simulink model "mfordmodel_v1"  (R2023a)
settings: Solver=ode45  StartTime=0.0  StopTime=10.0  RelTol=1e-3  EnableMultiTasking=on
undefined symbols (not defined in the file): ABV_RATIO_SW, AC_OFF_DLY, ACLOD, AUTO_TRNS_SW, BRAKE_DNDT_X, BZZRPM, BZZRPM_ALT, BZZTM, BZZTM_ALT, CMD_LITOFF, CMD_STABLE, CO_ST_ECT__A, COOL_BASE, DAS_BKDLY_A, DAS_CNT, DAS_CTDLY, DAS_LC_SW__A, DASCLP_5INH, DASCTL, DASMHYST, DASMPH, DEBYCP, DES_BASE, DPNEU_MUL, DSDRPM_DN_TC, DSDRPM_OFF, DSDRPM_UP_TC, EDF_DELAY, EDFHP, ETC_CL_TP, ETC_HP, GR_CM_CREEP, HCAM_ACT_CLP, HEDFHP, HEDFRPM, HICAM_PS, IAC_CAL_SW, IAC_ER_TM1, IAC_ER_TM2, IAC_ER_TM4, IAC_HI_LIM__A, IAC_ISFL_OBD, IAC_KAM_SW, IAC_LO_LIM__A, IAC_MON_TM, IAC_OT_REQ, IAC_RUN_TM, IAC_TP_OBD, IAC_TR_DAS, IAC_TST_DC, ID_DAS__A, ID_NOVS__A, IDVS_CH__A, IDVS_SL__A, IPSI_SW, IPSIDLY, IS_DRBASE__A, IS_DRBASE_A__A, IS_NUBASE__A, IS_NUBASE_A__A ... (+35)
libraries: simulink x2
(part 6 of 12)

== system mfordmodel_v1/iac_v04_001_001/activate_desired_rpm/hicam_rpm_request/isadd_ramp/CONSTANT ==
  Constant : Constant  Value=const
  Out : Outport
  wires:
  Constant/1 -> Out/1

== system mfordmodel_v1/iac_v04_001_001/activate_desired_rpm/hicam_rpm_request/isadd_ramp/ROLAV_TC_in_DT_in ==
  note: Using the first two terms of the series expansion:
      |
      |                     x                     x2
      |                                e   =  1  +  x  +  --  + ......
      |                                           2!
      |
      |       Simplifying, the exponential "f" becomes:
      |
      |                  - (FK_TMR/TC)              1
      |           f  =  1  -  e                    =  1  -  -------------  =  . . .
      |                                                    (FK_TMR/TC)
      |                           e
      |
      |                              1                      1
      |          f  =  1  -  ---------------------------------  =    ------------------- .
      |                                  1 + (FK_TMR / TC)       1 + (TC / FK_TMR)
  note: - (FK_TMR/TC)
      |                                    f  =  1  -  e
      |
      |       Where "f" is called the filter constant in the difference equation:
      |
      |                    new_average = f * new_value + (1 - f) * old_average
  note: new_average = [ (sample_interval)/(sample_interval + time_constant) ] * (new_value - old_ave) + old_ave
  new_value : Inport
  Tau : Inport  Port=2
  old_ave : Inport  Port=3
  delta_time : Inport  Port=4
  Elementary Math : Math  Operator=reciprocal  SignedPower=on
  Product : Product  Inputs=3  InputSameDT=on  RndMeth=Zero  SaturateOnIntegerOverflow=on  OutDataTypeStr=Inherit: Same as first input
  Sum : Sum  Inputs=-+  InputSameDT=on  SaturateOnIntegerOverflow=on  OutDataTypeStr=Inherit: Same as first input
  Sum1 : Sum  InputSameDT=on  SaturateOnIntegerOverflow=on  OutDataTypeStr=Inherit: Same as first input
  Sum2 : Sum  InputSameDT=on  SaturateOnIntegerOverflow=on  OutDataTypeStr=Inherit: Same as first input
  new_ave : Outport
  wires:
  delta_time/1 -> Product/2, Sum1/1
  Tau/1 -> Sum1/2
  Sum2/1 -> new_ave/1
  old_ave/1 -> Sum2/1, Sum/1
  Product/1 -> Sum2/2
  Sum/1 -> Product/1
  Elementary Math/1 -> Product/3
  Sum1/1 -> Elementary Math/1
  new_value/1 -> Sum/2

== system mfordmodel_v1/iac_v04_001_001/iac_executive/fault_code_setting/TIMER_DT_in/Time Calculator ==
  note: Timer Control calls the counters 'delta_time' and 'timer_calculation'
      | after using the flags 'increment_flag' and 'decrement_flag'
      | to determine the direction of the timer.
  note: Increment, hold,
      | or decrement
  note: Resets timer
      | to 'reset_value'
  note: Calculates time
      | between cycles.
      | Activated every cycle.
  note: Calculates timer value.
      | Activated only when
      | counting up or down.
  count_direction : Inport
  reset_val : Inport  Port=2
  do_delta_time : Inport  Port=3
  do_timer : Inport  Port=4
  reset_value : Inport  Port=5
  delta time : Inport  Port=6
  From : From
  Goto : Goto
  delta_time : Subsystem  TreatAsAtomicUnit=on
  timer_calculation : Subsystem  TreatAsAtomicUnit=on
  timer : Outport
  wires:
  do_delta_time/1 -> delta_time/Trigger  "do_delta_time"
  delta_time/1(delta_time) -> Goto/1  "delta_time"
  count_direction/1 -> delta_time/1(count_direction)  "count_direction"
  timer_calculation/1(timer) -> timer/1  "timer"
  From/1 -> timer_calculation/3(delta_time)  "delta_time"
  do_timer/1 -> timer_calculation/Trigger  "do_timer"
  reset_val/1 -> timer_calculation/2(reset_flag)  "reset_flag"
  reset_value/1 -> timer_calculation/1(reset_value)  "reset_value"
  delta time/1 -> delta_time/2(count_direction1)  "delta_time"

== system mfordmodel_v1/iac_v04_001_001/iac_executive/misc_calcs/TIMER_DT_in/Time Calculator ==
  note: Timer Control calls the counters 'delta_time' and 'timer_calculation'
      | after using the flags 'increment_flag' and 'decrement_flag'
      | to determine the direction of the timer.
  note: Increment, hold,
      | or decrement
  note: Resets timer
      | to 'reset_value'
  note: Calculates time
      | between cycles.
      | Activated every cycle.
  note: Calculates timer value.
      | Activated only when
      | counting up or down.
  count_direction : Inport
  reset_val : Inport  Port=2
  do_delta_time : Inport  Port=3
  do_timer : Inport  Port=4
  reset_value : Inport  Port=5
  delta time : Inport  Port=6
  From : From
  Goto : Goto
  delta_time : Subsystem  TreatAsAtomicUnit=on
  timer_calculation : Subsystem  TreatAsAtomicUnit=on
  timer : Outport
  wires:
  do_delta_time/1 -> delta_time/Trigger  "do_delta_time"
  delta_time/1(delta_time) -> Goto/1  "delta_time"
  count_direction/1 -> delta_time/1(count_direction)  "count_direction"
  timer_calculation/1(timer) -> timer/1  "timer"
  From/1 -> timer_calculation/3(delta_time)  "delta_time"
  do_timer/1 -> timer_calculation/Trigger  "do_timer"
  reset_val/1 -> timer_calculation/2(reset_flag)  "reset_flag"
  reset_value/1 -> timer_calculation/1(reset_value)  "reset_value"
  delta time/1 -> delta_time/2(count_direction1)  "delta_time"

== system mfordmodel_v1/iac_v04_001_001/iac_executive/misc_calcs/dndt_calc/ROLAV_TC_DT_in ==
  note: Using the first two terms of the series expansion:
      |
      |                     x                     x2
      |                                e   =  1  +  x  +  --  + ......
      |                                           2!
      |
      |       Simplifying, the exponential "f" becomes:
      |
      |                  - (FK_TMR/TC)              1
      |           f  =  1  -  e                    =  1  -  -------------  =  . . .
      |                                                    (FK_TMR/TC)
      |                           e
      |
      |                              1                      1
      |          f  =  1  -  ---------------------------------  =    ------------------- .
      |                                  1 + (FK_TMR / TC)       1 + (TC / FK_TMR)
  note: - (FK_TMR/TC)
      |                                    f  =  1  -  e
      |
      |       Where "f" is called the filter constant in the difference equation:
      |
      |                    new_average = f * new_value + (1 - f) * old_average
  note: new_average = [ (sample_interval)/(sample_interval + time_constant) ] * (new_value - old_ave) + old_ave
  new_value : Inport
  old_ave : Inport  Port=2
  delta_time : Inport  Port=3
  Elementary Math : Math  Operator=reciprocal  SignedPower=on
  Product : Product  Inputs=3  InputSameDT=on  RndMeth=Zero  SaturateOnIntegerOverflow=on  OutDataTypeStr=Inherit: Same as first input
  Sum : Sum  Inputs=-+  InputSameDT=on  SaturateOnIntegerOverflow=on  OutDataTypeStr=Inherit: Same as first input
  Sum1 : Sum  InputSameDT=on  SaturateOnIntegerOverflow=on  OutDataTypeStr=Inherit: Same as first input
  Sum2 : Sum  InputSameDT=on  SaturateOnIntegerOverflow=on  OutDataTypeStr=Inherit: Same as first input
  Time Constant : Constant  Value=tc
  new_ave : Outport
  wires:
  Time Constant/1 -> Sum1/2
  Sum2/1 -> new_ave/1
  old_ave/1 -> Sum2/1, Sum/1
  Product/1 -> Sum2/2
  Sum/1 -> Product/1
  Elementary Math/1 -> Product/3
  Sum1/1 -> Elementary Math/1
  new_value/1 -> Sum/2
  delta_time/1 -> Product/2, Sum1/1

== system mfordmodel_v1/iac_v04_001_001/iac_executive/mode_control/crank_mode/crank_calcs ==
  ml_flow_sel_sw : Inport
  tcstrt : Inport  Port=2
  ratch : Inport  Port=3
  do_crank_calcs : TriggerPort  TriggerType=function-call  VariantControl=(inherit)
  Constant : Constant  Value=0.0
  Constant1 : Constant  Value=0.0
  Constant2 : Constant
  Gain : Gain  SaturateOnIntegerOverflow=on  OutDataTypeStr=Inherit: Same as input  ParamDataTypeStr=Inherit: Same as input
  ISCFLG_DASHPOT_PREPOSITION : Constant  Value=0
  Multiport Switch9 : MultiPortSwitch  Inputs=2
  lookup_2d FN818 : Subsystem  mask(2-D, piece-wise, linear interpolation){CAL_FUNC=FNCRANK_PPM}
      mask prompts: CAL_FUNC "Calibration function name"
      mask help:
      | Performs piece-wise linear interpolation.
      |
      | Output is NOT extrapolated beyond the input range.  If the input value presented to the block lies outside the range specified in the block's parameter, then the value is treated as though it has the value of the nearest value in the range.
      mask init: same as mfordmodel_v1/iac_v04_001_001/activate_desired_rpm/rpm_calcs/lookup_2d
      mask Help:
      | Enter the name of the calibration function.
      | (e.g. EGM_VA_ECT_MULT)
      mask Display:
      | fprintf('%s',CAL_FUNC);
      | plot(calfunc.X,calfunc.Y,max_x*1.05,max_y*1.05,min_x,min_y);
  abv_ratio : Outport  InitialOutput=[0]
  abv_flowrate : Outport  Port=2  InitialOutput=[0]
  hcamfg : Outport  Port=3  InitialOutput=[0]
  iscflg : Outport  Port=4  InitialOutput=[0]
  dstpbr : Outport  Port=5  InitialOutput=[0]
  wires:
  Gain/1 -> dstpbr/1  "dstpbr"
  ratch/1 -> Gain/1
  ISCFLG_DASHPOT_PREPOSITION/1 -> iscflg/1  "iscflg"
  Constant2/1 -> hcamfg/1  "hcamfg"
  Multiport Switch9/1 -> abv_flowrate/1  "abv_flowrate"
  ml_flow_sel_sw/1 -> Multiport Switch9/1
  lookup_2d FN818/1(Out1) -> Multiport Switch9/2
  tcstrt/1 -> lookup_2d FN818/1(In1)
  Constant1/1 -> Multiport Switch9/3
  Constant/1 -> abv_ratio/1  "abv_ratio"

== system mfordmodel_v1/iac_v04_001_001/iac_executive/mode_control/external_override_mode/flowrate_set ==
  ml_flow_sel_sw : Inport
  abv_flowrate_osc : Inport  Port=2
  abv_flowrate_in : Inport  Port=3
  abv_ratio_in : Inport  Port=4
  do_flowrate_set : TriggerPort  TriggerType=function-call  VariantControl=(inherit)
  Constant4 : Constant  Value=15.99976
  Constant5 : Constant  Value=0.0
  Constant6 : Constant  Value=0.0
  Multiport Switch : MultiPortSwitch  Inputs=4
  Multiport Switch1 : MultiPortSwitch  Inputs=4
  abv_flowrate : Outport
  abv_ratio : Outport  Port=2
  wires:
  abv_ratio_in/1 -> Multiport Switch1/5
  abv_flowrate_in/1 -> Multiport Switch/5
  Constant6/1 -> Multiport Switch1/4, Multiport Switch1/3, Multiport Switch1/2
  ml_flow_sel_sw/1 -> Multiport Switch/1, Multiport Switch1/1
  Multiport Switch1/1 -> abv_ratio/1  "abv_ratio"
  Constant5/1 -> Multiport Switch/4
  Constant4/1 -> Multiport Switch/3
  abv_flowrate_osc/1 -> Multiport Switch/2
  Multiport Switch/1 -> abv_flowrate/1  "abv_flowrate"

== system mfordmodel_v1/iac_v04_001_001/iac_executive/mode_control/external_override_mode/substitute ==
  note: For now, just pass through the value.
      | Later, the substitution logic will be added.
  OSC_in : Inport
  do_substitute : TriggerPort  TriggerType=function-call  VariantControl=(inherit)
  Gain : Gain  SaturateOnIntegerOverflow=on  OutDataTypeStr=Inherit: Same as input  ParamDataTypeStr=Inherit: Same as input
  OSC_out : Outport
  wires:
  Gain/1 -> OSC_out/1
  OSC_in/1 -> Gain/1

== system mfordmodel_v1/iac_v04_001_001/iac_executive/mode_control/failure_mode/CONSTANT1 ==
  Constant : Constant  Value=const
  Out : Outport
  wires:
  Constant/1 -> Out/1

== system mfordmodel_v1/iac_v04_001_001/iac_executive/runup_flag_timer/TIMER_DT_in/Time Calculator ==
  note: Timer Control calls the counters 'delta_time' and 'timer_calculation'
      | after using the flags 'increment_flag' and 'decrement_flag'
      | to determine the direction of the timer.
  note: Increment, hold,
      | or decrement
  note: Resets timer
      | to 'reset_value'
  note: Calculates time
      | between cycles.
      | Activated every cycle.
  note: Calculates timer value.
      | Activated only when
      | counting up or down.
  count_direction : Inport
  reset_val : Inport  Port=2
  do_delta_time : Inport  Port=3
  do_timer : Inport  Port=4
  reset_value : Inport  Port=5
  delta time : Inport  Port=6
  From : From
  Goto : Goto
  delta_time : Subsystem  TreatAsAtomicUnit=on
  timer_calculation : Subsystem  TreatAsAtomicUnit=on
  timer : Outport
  wires:
  do_delta_time/1 -> delta_time/Trigger  "do_delta_time"
  delta_time/1(delta_time) -> Goto/1  "delta_time"
  count_direction/1 -> delta_time/1(count_direction)  "count_direction"
  timer_calculation/1(timer) -> timer/1  "timer"
  From/1 -> timer_calculation/3(delta_time)  "delta_time"
  do_timer/1 -> timer_calculation/Trigger  "do_timer"
  reset_val/1 -> timer_calculation/2(reset_flag)  "reset_flag"
  reset_value/1 -> timer_calculation/1(reset_value)  "reset_value"
  delta time/1 -> delta_time/2(count_direction1)  "delta_time"

== system mfordmodel_v1/iac_v04_001_001/normal_mode/activate_feedforward/ac_ppm_tmr/Time Calculator ==
  note: Calculates timer value.
      | Activated only when
      | counting up or down.
  note: Calculates time
      | between cycles.
      | Activated every cycle.
  note: Resets timer
      | to 'reset_value'
  note: Increment, hold,
      | or decrement
  note: Timer Control calls the counters 'delta_time' and 'timer_calculation'
      | after using the flags 'increment_flag' and 'decrement_flag'
      | to determine the direction of the timer.
  note: timer14/TIMER/Time Calculator
  count_direction : Inport
  reset_val : Inport  Port=2
  do_delta_time : Inport  Port=3
  do_timer : Inport  Port=4
  reset_value : Inport  Port=5
  From : From
  Goto : Goto
  delta_time : Subsystem  TreatAsAtomicUnit=on
  timer_calculation : Subsystem  TreatAsAtomicUnit=on
  timer : Outport
  wires:
  reset_value/1 -> timer_calculation/1(reset_value)  "reset_value"
  reset_val/1 -> timer_calculation/2(reset_flag)  "reset_flag"
  do_timer/1 -> timer_calculation/Trigger  "do_timer"
  From/1 -> timer_calculation/3(delta_time)  "delta_time"
  timer_calculation/1(timer) -> timer/1  "timer"
  count_direction/1 -> delta_time/1(count_direction)  "count_direction"
  delta_time/1(delta_time) -> Goto/1  "delta_time"
  do_delta_time/1 -> delta_time/Trigger  "do_delta_time"

== system mfordmodel_v1/iac_v04_001_001/normal_mode/activate_feedforward/desmaf_pre_calc/   ==
  Constant : Constant  Value=const
  Out : Outport
  wires:
  Constant/1 -> Out/1

== system mfordmodel_v1/iac_v04_001_001/normal_mode/activate_feedforward/desmaf_pre_calc/  2 ==
  Constant : Constant  Value=const
  Out : Outport
  wires:
  Constant/1 -> Out/1

== system mfordmodel_v1/iac_v04_001_001/normal_mode/activate_feedforward/desmaf_pre_calc/1 ==
  Constant : Constant  Value=const
  Out : Outport
  wires:
  Constant/1 -> Out/1

== system mfordmodel_v1/iac_v04_001_001/normal_mode/activate_feedforward/desmaf_pre_calc/3 ==
  Constant : Constant  Value=const
  Out : Outport
  wires:
  Constant/1 -> Out/1

== system mfordmodel_v1/iac_v04_001_001/normal_mode/activate_feedforward/desmaf_pre_calc/FN018E2 ==
  In1 : Inport
  Look-Up Table1 : Lookup  InputValues=calfunc.X  Table=calfunc.Y
  Saturation1 : Saturate  UpperLimit=max_x  LowerLimit=min_x
  Out1 : Outport
  wires:
  In1/1 -> Saturation1/1
  Saturation1/1 -> Look-Up Table1/1
  Look-Up Table1/1 -> Out1/1

== system mfordmodel_v1/iac_v04_001_001/normal_mode/activate_feedforward/desmaf_pre_calc/FN020C3 ==
  In1 : Inport
  Look-Up Table1 : Lookup  InputValues=calfunc.X  Table=calfunc.Y
  Saturation1 : Saturate  UpperLimit=max_x  LowerLimit=min_x
  Out1 : Outport
  wires:
  In1/1 -> Saturation1/1
  Saturation1/1 -> Look-Up Table1/1
  Look-Up Table1/1 -> Out1/1

== system mfordmodel_v1/iac_v04_001_001/normal_mode/activate_feedforward/desmaf_pre_calc/FN1862AD ==
  X : Inport
  Y : Inport  Port=2
  Look-Up Table (2-D) : Lookup2D  RowIndex=caltable.Y  ColumnIndex=caltable.X  Table=caltable.Z
  Saturation1 : Saturate  UpperLimit=max_x  LowerLimit=min_x
  Saturation2 : Saturate  UpperLimit=max_y  LowerLimit=min_y
  Z : Outport
  wires:
  Look-Up Table (2-D)/1 -> Z/1  "z"
  Y/1 -> Saturation2/1
  X/1 -> Saturation1/1
  Saturation1/1 -> Look-Up Table (2-D)/2
  Saturation2/1 -> Look-Up Table (2-D)/1

== system mfordmodel_v1/iac_v04_001_001/normal_mode/activate_feedforward/desmaf_pre_calc/FN1862AN ==
  X : Inport
  Y : Inport  Port=2
  Look-Up Table (2-D) : Lookup2D  RowIndex=caltable.Y  ColumnIndex=caltable.X  Table=caltable.Z
  Saturation1 : Saturate  UpperLimit=max_x  LowerLimit=min_x
  Saturation2 : Saturate  UpperLimit=max_y  LowerLimit=min_y
  Z : Outport
  wires:
  Look-Up Table (2-D)/1 -> Z/1  "z"
  Y/1 -> Saturation2/1
  X/1 -> Saturation1/1
  Saturation1/1 -> Look-Up Table (2-D)/2
  Saturation2/1 -> Look-Up Table (2-D)/1

== system mfordmodel_v1/iac_v04_001_001/normal_mode/activate_feedforward/desmaf_pre_calc/FN803 ==
  In1 : Inport
  Look-Up Table1 : Lookup  InputValues=calfunc.X  Table=calfunc.Y
  Saturation1 : Saturate  UpperLimit=max_x  LowerLimit=min_x
  Out1 : Outport
  wires:
  In1/1 -> Saturation1/1
  Saturation1/1 -> Look-Up Table1/1
  Look-Up Table1/1 -> Out1/1

== system mfordmodel_v1/iac_v04_001_001/normal_mode/activate_feedforward/desmaf_pre_calc/FN806 ==
  In1 : Inport
  Look-Up Table1 : Lookup  InputValues=calfunc.X  Table=calfunc.Y
  Saturation1 : Saturate  UpperLimit=max_x  LowerLimit=min_x
  Out1 : Outport
  wires:
  In1/1 -> Saturation1/1
  Saturation1/1 -> Look-Up Table1/1
  Look-Up Table1/1 -> Out1/1

== system mfordmodel_v1/iac_v04_001_001/normal_mode/activate_feedforward/desmaf_pre_calc/FN855 ==
  In1 : Inport
  Look-Up Table1 : Lookup  InputValues=calfunc.X  Table=calfunc.Y
  Saturation1 : Saturate  UpperLimit=max_x  LowerLimit=min_x
  Out1 : Outport
  wires:
  In1/1 -> Saturation1/1
  Saturation1/1 -> Look-Up Table1/1
  Look-Up Table1/1 -> Out1/1

== system mfordmodel_v1/iac_v04_001_001/normal_mode/activate_feedforward/desmaf_pre_calc/FN875HD ==
  In1 : Inport
  Look-Up Table1 : Lookup  InputValues=calfunc.X  Table=calfunc.Y
  Saturation1 : Saturate  UpperLimit=max_x  LowerLimit=min_x
  Out1 : Outport
  wires:
  In1/1 -> Saturation1/1
  Saturation1/1 -> Look-Up Table1/1
  Look-Up Table1/1 -> Out1/1

== system mfordmodel_v1/iac_v04_001_001/normal_mode/activate_feedforward/desmaf_pre_calc/FN875HN ==
  In1 : Inport
  Look-Up Table1 : Lookup  InputValues=calfunc.X  Table=calfunc.Y
  Saturation1 : Saturate  UpperLimit=max_x  LowerLimit=min_x
  Out1 : Outport
  wires:
  In1/1 -> Saturation1/1
  Saturation1/1 -> Look-Up Table1/1
  Look-Up Table1/1 -> Out1/1

== system mfordmodel_v1/iac_v04_001_001/normal_mode/activate_feedforward/desmaf_pre_calc/FN885TE ==
  In1 : Inport
  Look-Up Table1 : Lookup  InputValues=calfunc.X  Table=calfunc.Y
  Saturation1 : Saturate  UpperLimit=max_x  LowerLimit=min_x
  Out1 : Outport
  wires:
  In1/1 -> Saturation1/1
  Saturation1/1 -> Look-Up Table1/1
  Look-Up Table1/1 -> Out1/1

== system mfordmodel_v1/iac_v04_001_001/normal_mode/activate_feedforward/desmaf_pre_calc/FN887ME ==
  In1 : Inport
  Look-Up Table1 : Lookup  InputValues=calfunc.X  Table=calfunc.Y
  Saturation1 : Saturate  UpperLimit=max_x  LowerLimit=min_x
  Out1 : Outport
  wires:
  In1/1 -> Saturation1/1
  Saturation1/1 -> Look-Up Table1/1
  Look-Up Table1/1 -> Out1/1

== system mfordmodel_v1/iac_v04_001_001/normal_mode/activate_feedforward/desmaf_pre_calc/FN887VC ==
  In1 : Inport
  Look-Up Table1 : Lookup  InputValues=calfunc.X  Table=calfunc.Y
  Saturation1 : Saturate  UpperLimit=max_x  LowerLimit=min_x
  Out1 : Outport
  wires:
  In1/1 -> Saturation1/1
  Saturation1/1 -> Look-Up Table1/1
  Look-Up Table1/1 -> Out1/1

== system mfordmodel_v1/iac_v04_001_001/normal_mode/activate_feedforward/desmaf_pre_calc/FN896 ==
  In1 : Inport
  Look-Up Table1 : Lookup  InputValues=calfunc.X  Table=calfunc.Y
  Saturation1 : Saturate  UpperLimit=max_x  LowerLimit=min_x
  Out1 : Outport
  wires:
  In1/1 -> Saturation1/1
  Saturation1/1 -> Look-Up Table1/1
  Look-Up Table1/1 -> Out1/1

== system mfordmodel_v1/iac_v04_001_001/normal_mode/activate_feedforward/desmaf_pre_calc/FN896A ==
  In1 : Inport
  Look-Up Table1 : Lookup  InputValues=calfunc.X  Table=calfunc.Y
  Saturation1 : Saturate  UpperLimit=max_x  LowerLimit=min_x
  Out1 : Outport
  wires:
  In1/1 -> Saturation1/1
  Saturation1/1 -> Look-Up Table1/1
  Look-Up Table1/1 -> Out1/1

== system mfordmodel_v1/iac_v04_001_001/normal_mode/activate_feedforward/desmaf_pre_calc/FNLOSS_D_PPM ==
  In1 : Inport
  Look-Up Table1 : Lookup  InputValues=calfunc.X  Table=calfunc.Y
  Saturation1 : Saturate  UpperLimit=max_x  LowerLimit=min_x
  Out1 : Outport
  wires:
  In1/1 -> Saturation1/1
  Saturation1/1 -> Look-Up Table1/1
  Look-Up Table1/1 -> Out1/1

== system mfordmodel_v1/iac_v04_001_001/normal_mode/activate_feedforward/desmaf_pre_calc/FNLOSS_N_PPM ==
  In1 : Inport
  Look-Up Table1 : Lookup  InputValues=calfunc.X  Table=calfunc.Y
  Saturation1 : Saturate  UpperLimit=max_x  LowerLimit=min_x
  Out1 : Outport
  wires:
  In1/1 -> Saturation1/1
  Saturation1/1 -> Look-Up Table1/1
  Look-Up Table1/1 -> Out1/1

== system mfordmodel_v1/iac_v04_001_001/normal_mode/activate_feedforward/desmaf_pre_calc/ROLAV_TC_DT_in ==
  note: Using the first two terms of the series expansion:
      |
      |                     x                     x2
      |                                e   =  1  +  x  +  --  + ......
      |                                           2!
      |
      |       Simplifying, the exponential "f" becomes:
      |
      |                  - (FK_TMR/TC)              1
      |           f  =  1  -  e                    =  1  -  -------------  =  . . .
      |                                                    (FK_TMR/TC)
      |                           e
      |
      |                              1                      1
      |          f  =  1  -  ---------------------------------  =    ------------------- .
      |                                  1 + (FK_TMR / TC)       1 + (TC / FK_TMR)
  note: - (FK_TMR/TC)
      |                                    f  =  1  -  e
      |
      |       Where "f" is called the filter constant in the difference equation:
      |
      |                    new_average = f * new_value + (1 - f) * old_average
  note: new_average = [ (sample_interval)/(sample_interval + time_constant) ] * (new_value - old_ave) + old_ave
  new_value : Inport
  old_ave : Inport  Port=2
  delta_time : Inport  Port=3
  Elementary Math : Math  Operator=reciprocal  SignedPower=on
  Product : Product  Inputs=3  InputSameDT=on  RndMeth=Zero  SaturateOnIntegerOverflow=on  OutDataTypeStr=Inherit: Same as first input
  Sum : Sum  Inputs=-+  InputSameDT=on  SaturateOnIntegerOverflow=on  OutDataTypeStr=Inherit: Same as first input
  Sum1 : Sum  InputSameDT=on  SaturateOnIntegerOverflow=on  OutDataTypeStr=Inherit: Same as first input
  Sum2 : Sum  InputSameDT=on  SaturateOnIntegerOverflow=on  OutDataTypeStr=Inherit: Same as first input
  Time Constant : Constant  Value=tc
  new_ave : Outport
  wires:
  Time Constant/1 -> Sum1/2
  Sum2/1 -> new_ave/1
  old_ave/1 -> Sum2/1, Sum/1
  Product/1 -> Sum2/2
  Sum/1 -> Product/1
  Elementary Math/1 -> Product/3
  Sum1/1 -> Elementary Math/1
  new_value/1 -> Sum/2
  delta_time/1 -> Product/2, Sum1/1

== system mfordmodel_v1/iac_v04_001_001/normal_mode/activate_feedforward/desmaf_pre_calc/lookup_2d ==
  In1 : Inport
  Look-Up Table1 : Lookup  InputValues=calfunc.X  Table=calfunc.Y
  Saturation1 : Saturate  UpperLimit=max_x  LowerLimit=min_x
  Out1 : Outport
  wires:
  In1/1 -> Saturation1/1
  Saturation1/1 -> Look-Up Table1/1
  Look-Up Table1/1 -> Out1/1

== system mfordmodel_v1/iac_v04_001_001/normal_mode/activate_kam/iac_kam_tmr/Time Calculator ==
  note: Calculates timer value.
      | Activated only when
      | counting up or down.
  note: Calculates time
      | between cycles.
      | Activated every cycle.
  note: Resets timer
      | to 'reset_value'
  note: Increment, hold,
      | or decrement
  note: Timer Control calls the counters 'delta_time' and 'timer_calculation'
      | after using the flags 'increment_flag' and 'decrement_flag'
      | to determine the direction of the timer.
  note: timer14/TIMER/Time Calculator
  count_direction : Inport
  reset_val : Inport  Port=2
  do_delta_time : Inport  Port=3
  do_timer : Inport  Port=4
  reset_value : Inport  Port=5
  From : From
  Goto : Goto
  delta_time : Subsystem  TreatAsAtomicUnit=on
  timer_calculation : Subsystem  TreatAsAtomicUnit=on
  timer : Outport
  wires:
  reset_value/1 -> timer_calculation/1(reset_value)  "reset_value"
  reset_val/1 -> timer_calculation/2(reset_flag)  "reset_flag"
  do_timer/1 -> timer_calculation/Trigger  "do_timer"
  From/1 -> timer_calculation/3(delta_time)  "delta_time"
  timer_calculation/1(timer) -> timer/1  "timer"
  count_direction/1 -> delta_time/1(count_direction)  "count_direction"
  delta_time/1(delta_time) -> Goto/1  "delta_time"
  do_delta_time/1 -> delta_time/Trigger  "do_delta_time"

== system mfordmodel_v1/iac_v04_001_001/normal_mode/activate_kam/isckam_clear/CONSTANT1 ==
  Constant : Constant  Value=const
  Out : Outport
  wires:
  Constant/1 -> Out/1

== system mfordmodel_v1/iac_v04_001_001/normal_mode/activate_kam/isckam_clear/CONSTANT2 ==
  Constant : Constant  Value=const
  Out : Outport
  wires:
  Constant/1 -> Out/1

== system mfordmodel_v1/iac_v04_001_001/normal_mode/activate_kam/isckam_clear/CONSTANT3 ==
  Constant : Constant  Value=const
  Out : Outport
  wires:
  Constant/1 -> Out/1

== system mfordmodel_v1/iac_v04_001_001/normal_mode/activate_kam/isckam_clear/CONSTANT4 ==
  Constant : Constant  Value=const
  Out : Outport
  wires:
  Constant/1 -> Out/1

== system mfordmodel_v1/iac_v04_001_001/normal_mode/activate_kam/isckam_clear/CONSTANT5 ==
  Constant : Constant  Value=const
  Out : Outport
  wires:
  Constant/1 -> Out/1

== system mfordmodel_v1/iac_v04_001_001/normal_mode/activate_kam/isckam_clear/CONSTANT6 ==
  Constant : Constant  Value=const
  Out : Outport
  wires:
  Constant/1 -> Out/1

== system mfordmodel_v1/iac_v04_001_001/normal_mode/activate_kam/isckam_clear/CONSTANT7 ==
  Constant : Constant  Value=const
  Out : Outport
  wires:
  Constant/1 -> Out/1

== system mfordmodel_v1/iac_v04_001_001/normal_mode/activate_kam/isckam_clear/CONSTANT8 ==
  Constant : Constant  Value=const
  Out : Outport
  wires:
  Constant/1 -> Out/1

== system mfordmodel_v1/iac_v04_001_001/normal_mode/activate_kam/update_pids/CONSTANT1 ==
  Constant : Constant  Value=const
  Out : Outport
  wires:
  Constant/1 -> Out/1

== system mfordmodel_v1/iac_v04_001_001/normal_mode/activate_kam/update_pids/pid ==
  data : Inport
  ctrl : Inport  Port=2
  Terminator : Terminator
  Terminator1 : Terminator
  wires:
  ctrl/1 -> Terminator1/1
  data/1 -> Terminator/1

== system mfordmodel_v1/iac_v04_001_001/normal_mode/activate_kam/update_pids/pid1 ==
  data : Inport
  ctrl : Inport  Port=2
  Terminator : Terminator
  Terminator1 : Terminator
  wires:
  ctrl/1 -> Terminator1/1
  data/1 -> Terminator/1

== system mfordmodel_v1/iac_v04_001_001/normal_mode/activate_kam/update_pids/pid2 ==
  data : Inport
  ctrl : Inport  Port=2
  Terminator : Terminator
  Terminator1 : Terminator
  wires:
  ctrl/1 -> Terminator1/1
  data/1 -> Terminator/1

== system mfordmodel_v1/iac_v04_001_001/normal_mode/activate_kam/update_pids/pid3 ==
  data : Inport
  ctrl : Inport  Port=2
  Terminator : Terminator
  Terminator1 : Terminator
  wires:
  ctrl/1 -> Terminator1/1
  data/1 -> Terminator/1

== system mfordmodel_v1/iac_v04_001_001/normal_mode/activate_normal_mode/dstpbr_calc/CONSTANT ==
  Constant : Constant  Value=const
  Out : Outport
  wires:
  Constant/1 -> Out/1

== system mfordmodel_v1/iac_v04_001_001/normal_mode/activate_normal_mode/dstpbr_calc/CONSTANT1 ==
  Constant : Constant  Value=const
  Out : Outport
  wires:
  Constant/1 -> Out/1

== system mfordmodel_v1/iac_v04_001_001/normal_mode/activate_normal_mode/dstpbr_calc/ROLAV_TC_in_DT_in ==
  note: Using the first two terms of the series expansion:
      |
      |                     x                     x2
      |                                e   =  1  +  x  +  --  + ......
      |                                           2!
      |
      |       Simplifying, the exponential "f" becomes:
      |
      |                  - (FK_TMR/TC)              1
      |           f  =  1  -  e                    =  1  -  -------------  =  . . .
      |                                                    (FK_TMR/TC)
      |                           e
      |
      |                              1                      1
      |          f  =  1  -  ---------------------------------  =    ------------------- .
      |                                  1 + (FK_TMR / TC)       1 + (TC / FK_TMR)
  note: - (FK_TMR/TC)
      |                                    f  =  1  -  e
      |
      |       Where "f" is called the filter constant in the difference equation:
      |
      |                    new_average = f * new_value + (1 - f) * old_average
  note: new_average = [ (sample_interval)/(sample_interval + time_constant) ] * (new_value - old_ave) + old_ave
  new_value : Inport
  Tau : Inport  Port=2
  old_ave : Inport  Port=3
  delta_time : Inport  Port=4
  Elementary Math : Math  Operator=reciprocal  SignedPower=on
  Product : Product  Inputs=3  InputSameDT=on  RndMeth=Zero  SaturateOnIntegerOverflow=on  OutDataTypeStr=Inherit: Same as first input
  Sum : Sum  Inputs=-+  InputSameDT=on  SaturateOnIntegerOverflow=on  OutDataTypeStr=Inherit: Same as first input
  Sum1 : Sum  InputSameDT=on  SaturateOnIntegerOverflow=on  OutDataTypeStr=Inherit: Same as first input
  Sum2 : Sum  InputSameDT=on  SaturateOnIntegerOverflow=on  OutDataTypeStr=Inherit: Same as first input
  new_ave : Outport
  wires:
  delta_time/1 -> Product/2, Sum1/1
  Tau/1 -> Sum1/2
  Sum2/1 -> new_ave/1
  old_ave/1 -> Sum2/1, Sum/1
  Product/1 -> Sum2/2
  Sum/1 -> Product/1
  Elementary Math/1 -> Product/3
  Sum1/1 -> Elementary Math/1
  new_value/1 -> Sum/2

== system mfordmodel_v1/iac_v04_001_001/normal_mode/activate_normal_mode/ipsibr_clipping/ipsibr_clip ==
  note: Part of initialization Logic
  ml_max_clip : Inport
  ml_min_clip : Inport  Port=2
  ipsibr_kam : Inport  Port=3
  ml_limit_sw : Inport  Port=4
  ml_normal_init : Inport  Port=5
  do_ipsibr_clip : TriggerPort  TriggerType=function-call  VariantControl=(inherit)
  CONSTANT : Subsystem  mask(Constant){constant=PSIBRN}
      mask help: Constant Block. Will dispaly constant name and value on the icon of the block
      mask init:
      | if isletter(constant(1))
      |   const = evalin('base',constant);
      |   name = constant;
      | else
      |   const = str2num(constant);
      |   name = 'CONST';
      | end;
      mask Display: fprintf('%s = %.4f',name,const);
  CONSTANT1 : Subsystem  mask(Constant){constant=PSIBRM}
      mask help: Constant Block. Will dispaly constant name and value on the icon of the block
      mask init:
      | if isletter(constant(1))
      |   const = evalin('base',constant);
      |   name = constant;
      | else
      |   const = str2num(constant);
      |   name = 'CONST';
      | end;
      mask Display: fprintf('%s = %.4f',name,const);
  CONSTANT2 : Subsystem  mask(Constant){constant=IPSIMAX}
      mask help: Constant Block. Will dispaly constant name and value on the icon of the block
      mask init:
      | if isletter(constant(1))
      |   const = evalin('base',constant);
      |   name = constant;
      | else
      |   const = str2num(constant);
      |   name = 'CONST';
      | end;
      mask Display: fprintf('%s = %.4f',name,const);
  Constant : Constant  Value=0.0
  Constant1 : Constant  Value=0.0
  Constant2 : Constant  Value=0.0
  Gain : Gain  SaturateOnIntegerOverflow=on  OutDataTypeStr=Inherit: Same as input  ParamDataTypeStr=Inherit: Same as input
  Multiport Switch{6..9} (4 alike) : MultiPortSwitch  Inputs=2
  Terminator : Terminator
  VAR_SATURATION : Subsystem  mask(VARIABLE SATURATION){}
      mask help: This block will clip the input between the MIN and MAX values specified as inputs to the block. In addition a LIMIT_FLAG will be set to 1 if the input is currently being clipped.
      mask Display:
      | plot( [0.2 0.3 0.5 0.6], [0.2 0.2 0.8 0.8])
      | text(0.2, 0.05, 'min')
      | text(0.5, 0.95, 'max')
  ipsibr : Outport  InitialOutput=0
  ipsibr_fb : Outport  Port=2  InitialOutput=0
  wires:
  ml_limit_sw/1 -> Multiport Switch9/1
  Constant2/1 -> Multiport Switch9/3
  Multiport Switch9/1 -> VAR_SATURATION/2(INPUT)
  ipsibr_kam/1 -> Multiport Switch9/2
  Constant/1 -> Multiport Switch6/2
  ml_min_clip/1 -> Multiport Switch6/1
  CONSTANT/1(Out) -> Multiport Switch6/3
  Multiport Switch6/1 -> VAR_SATURATION/3(MIN)
  ml_max_clip/1 -> Multiport Switch7/1
  CONSTANT1/1(Out) -> Multiport Switch7/3
  CONSTANT2/1(Out) -> Multiport Switch7/2
  Multiport Switch7/1 -> VAR_SATURATION/1(MAX)
  VAR_SATURATION/2(LIMIT_FLAG) -> Terminator/1
  Gain/1 -> ipsibr_fb/1  "ipsibr_fb"
  Constant1/1 -> Multiport Switch8/2
  ml_normal_init/1 -> Multiport Switch8/1
  VAR_SATURATION/1(OUTPUT) -> Multiport Switch8/3  "ipsibr"
  Multiport Switch8/1 -> ipsibr/1, Gain/1  "ipsibr"

== system mfordmodel_v1/iac_v04_001_001/normal_mode/activate_normal_mode/normal_mode_fault_codes/iac_er_tmr1 ==
  note: Timer Control calls functions within the Time Calculator
      | after using the flags 'increment_flag' and 'decrement_flag'
      | to determine the direction of the timer.
  note: timer14/TIMER
  trig_time : Inport
  trig_reset : Inport  Port=2
  reset value : Inport  Port=3
  inc flag : Inport  Port=4
  dec flag : Inport  Port=5
  Event Triggers : Mux  Inputs=2
  Time Calculator : Subsystem
  Timer Control : Stateflow chart  TreatAsAtomicUnit=on
  timer : Outport
  wires:
  reset value/1 -> Time Calculator/5(reset_value)  "reset_value"
  trig_reset/1 -> Event Triggers/2  "trig_reset"
  trig_time/1 -> Event Triggers/1  "trig_timer"
  Event Triggers/1 -> Timer Control/Trigger
  Time Calculator/1(timer) -> timer/1  "timer"
  Timer Control/1(count_direction) -> Time Calculator/1(count_direction)  "count_direction"
  Timer Control/2(reset_flag) -> Time Calculator/2(reset_val)  "reset_flag"
  Timer Control/3(do_delta_time()) -> Time Calculator/3(do_delta_time)  "do_delta_time"
  Timer Control/4(do_timer()) -> Time Calculator/4(do_timer)  "do_timer"
  dec flag/1 -> Timer Control/2(decr_flag)  "decrement_flag"
  inc flag/1 -> Timer Control/1(incr_flag)  "increment_flag"

== system mfordmodel_v1/iac_v04_001_001/normal_mode/activate_normal_mode/normal_mode_fault_codes/iac_er_tmr2 ==
  note: Timer Control calls functions within the Time Calculator
      | after using the flags 'increment_flag' and 'decrement_flag'
      | to determine the direction of the timer.
  note: timer14/TIMER
  trig_time : Inport
  trig_reset : Inport  Port=2
  reset value : Inport  Port=3
  inc flag : Inport  Port=4
  dec flag : Inport  Port=5
  Event Triggers : Mux  Inputs=2
  Time Calculator : Subsystem
  Timer Control : Stateflow chart  TreatAsAtomicUnit=on
  timer : Outport
  wires:
  reset value/1 -> Time Calculator/5(reset_value)  "reset_value"
  trig_reset/1 -> Event Triggers/2  "trig_reset"
  trig_time/1 -> Event Triggers/1  "trig_timer"
  Event Triggers/1 -> Timer Control/Trigger
  Time Calculator/1(timer) -> timer/1  "timer"
  Timer Control/1(count_direction) -> Time Calculator/1(count_direction)  "count_direction"
  Timer Control/2(reset_flag) -> Time Calculator/2(reset_val)  "reset_flag"
  Timer Control/3(do_delta_time()) -> Time Calculator/3(do_delta_time)  "do_delta_time"
  Timer Control/4(do_timer()) -> Time Calculator/4(do_timer)  "do_timer"
  dec flag/1 -> Timer Control/2(decr_flag)  "decrement_flag"
  inc flag/1 -> Timer Control/1(incr_flag)  "increment_flag"

== system mfordmodel_v1/iac_v04_001_001/normal_mode/activate_normal_mode/normal_mode_fault_codes/iac_mon_tmr ==
  note: Timer Control calls functions within the Time Calculator
      | after using the flags 'increment_flag' and 'decrement_flag'
      | to determine the direction of the timer.
  note: timer14/TIMER
  trig_time : Inport
  trig_reset : Inport  Port=2
  reset value : Inport  Port=3
  inc flag : Inport  Port=4
  dec flag : Inport  Port=5
  Event Triggers : Mux  Inputs=2
  Time Calculator : Subsystem
  Timer Control : Stateflow chart  TreatAsAtomicUnit=on
  timer : Outport
  wires:
  reset value/1 -> Time Calculator/5(reset_value)  "reset_value"
  trig_reset/1 -> Event Triggers/2  "trig_reset"
  trig_time/1 -> Event Triggers/1  "trig_timer"
  Event Triggers/1 -> Timer Control/Trigger
  Time Calculator/1(timer) -> timer/1  "timer"
  Timer Control/1(count_direction) -> Time Calculator/1(count_direction)  "count_direction"
  Timer Control/2(reset_flag) -> Time Calculator/2(reset_val)  "reset_flag"
  Timer Control/3(do_delta_time()) -> Time Calculator/3(do_delta_time)  "do_delta_time"
  Timer Control/4(do_timer()) -> Time Calculator/4(do_timer)  "do_timer"
  dec flag/1 -> Timer Control/2(decr_flag)  "decrement_flag"
  inc flag/1 -> Timer Control/1(incr_flag)  "increment_flag"

== system mfordmodel_v1/iac_v04_001_001/normal_mode/activate_normal_mode/normal_mode_fault_codes/type1_fault_code ==
  trig_malfunction : Inport
  trig_clear_malf : Inport  Port=2
  Ground{,1..3} (4 alike) : Ground
  Mux : Mux  Inputs=2
  Mux1 : Mux  Inputs=5
  fault code_ctl : Stateflow chart  TreatAsAtomicUnit=on
  pxxxx : Outport
  wires:
  Ground1/1 -> Mux1/2  "pxxxstate"
  Ground2/1 -> Mux1/3  "pxxxmil_on"
  Ground3/1 -> Mux1/4  "pxxxfault"
  Ground/1 -> Mux1/1  "pxxxcnt"
  fault code_ctl/1(pxxxmalf) -> Mux1/5  "pxxxmalf"
  Mux1/1 -> pxxxx/1
  Mux/1 -> fault code_ctl/Trigger
  trig_clear_malf/1 -> Mux/2
  trig_malfunction/1 -> Mux/1

== system mfordmodel_v1/iac_v04_001_001/normal_mode/activate_normal_mode/normal_mode_fault_codes/type1_fault_code1 ==
  trig_malfunction : Inport
  trig_clear_malf : Inport  Port=2
  Ground{,1..3} (4 alike) : Ground
  Mux : Mux  Inputs=2
  Mux1 : Mux  Inputs=5
  fault code_ctl : Stateflow chart  TreatAsAtomicUnit=on
  pxxxx : Outport
  wires:
  Ground1/1 -> Mux1/2  "pxxxstate"
  Ground2/1 -> Mux1/3  "pxxxmil_on"
  Ground3/1 -> Mux1/4  "pxxxfault"
  Ground/1 -> Mux1/1  "pxxxcnt"
  fault code_ctl/1(pxxxmalf) -> Mux1/5  "pxxxmalf"
  Mux1/1 -> pxxxx/1
  Mux/1 -> fault code_ctl/Trigger
  trig_clear_malf/1 -> Mux/2
  trig_malfunction/1 -> Mux/1

== system mfordmodel_v1/iac_v04_001_001/normal_mode/activate_normal_mode/normal_mode_fault_codes/update_pids ==
  ipsibr : Inport
  ccm_iac_mon : Inport  Port=2
  iscflg : Inport  Port=3
  do_update_pids : TriggerPort  TriggerType=function-call  VariantControl=(inherit)
  " " : Subsystem  mask(PID){pid_cat=J2190, pid_number=0x095D, bit=BIT_15}
      mask prompts: pid_cat "PID Category"; pid_number "PID Number (e.g., 0x0C or 0x1123)"
      mask help:
      | Generic PID - used for J1979 (modes 1,2) and J2190.
      |
      | PID number is either 2 (J1979) or 4 ( J2190) digits, preceeded by 0x.
      |
      | BIT is selected from a pop-up list.
      |
      | CTRL is either CTRL_NONE (default) or your control parameter which enables/disables reporting of the PID.
      mask TypeOptions pid_cat: J1979MODE1 | J1979MODE2 | J1979MODE6 | J2190
      mask TypeOptions bit: BIT_NONE | BIT_00 | BIT_01 | BIT_02 | BIT_03 | BIT_04 | BIT_05 | BIT_06 | BIT_07 | BIT_08 | BIT_09 | BIT_10 | BIT_11 | BIT_12 | BIT_13 | BIT_14 | BIT_15 | BIT_16 | BIT_17 | BIT_18 | BIT_19 | BIT_20 | BIT_21 | BIT_22 | BIT_23 | BIT_24 | BIT_25 | BIT_26 | BIT_27 | BIT_28 | BIT_29 | BIT_30 | BIT_31
      mask Display: fprintf('%s\n%s\n%s',pid_cat,pid_number,bit);
  " 2" : Subsystem  mask(PID){pid_cat=J2190, pid_number=0x097A, bit=BIT_NONE}
      mask prompts: pid_cat "PID Category"; pid_number "PID Number (e.g., 0x0C or 0x1123)"
      mask help:
      | Generic PID - used for J1979 (modes 1,2) and J2190.
      |
      | PID number is either 2 (J1979) or 4 ( J2190) digits, preceeded by 0x.
      |
      | BIT is selected from a pop-up list.
      |
      | CTRL is either CTRL_NONE (default) or your control parameter which enables/disables reporting of the PID.
      mask TypeOptions pid_cat: J1979MODE1 | J1979MODE2 | J1979MODE6 | J2190
      mask TypeOptions bit: BIT_NONE | BIT_00 | BIT_01 | BIT_02 | BIT_03 | BIT_04 | BIT_05 | BIT_06 | BIT_07 | BIT_08 | BIT_09 | BIT_10 | BIT_11 | BIT_12 | BIT_13 | BIT_14 | BIT_15 | BIT_16 | BIT_17 | BIT_18 | BIT_19 | BIT_20 | BIT_21 | BIT_22 | BIT_23 | BIT_24 | BIT_25 | BIT_26 | BIT_27 | BIT_28 | BIT_29 | BIT_30 | BIT_31
      mask Display: fprintf('%s\n%s\n%s',pid_cat,pid_number,bit);
  " 3" : Subsystem  mask(PID){pid_cat=J2190, pid_number=0x097B, bit=BIT_NONE}
      mask prompts: pid_cat "PID Category"; pid_number "PID Number (e.g., 0x0C or 0x1123)"
      mask help:
      | Generic PID - used for J1979 (modes 1,2) and J2190.
      |
      | PID number is either 2 (J1979) or 4 ( J2190) digits, preceeded by 0x.
      |
      | BIT is selected from a pop-up list.
      |
      | CTRL is either CTRL_NONE (default) or your control parameter which enables/disables reporting of the PID.
      mask TypeOptions pid_cat: J1979MODE1 | J1979MODE2 | J1979MODE6 | J2190
      mask TypeOptions bit: BIT_NONE | BIT_00 | BIT_01 | BIT_02 | BIT_03 | BIT_04 | BIT_05 | BIT_06 | BIT_07 | BIT_08 | BIT_09 | BIT_10 | BIT_11 | BIT_12 | BIT_13 | BIT_14 | BIT_15 | BIT_16 | BIT_17 | BIT_18 | BIT_19 | BIT_20 | BIT_21 | BIT_22 | BIT_23 | BIT_24 | BIT_25 | BIT_26 | BIT_27 | BIT_28 | BIT_29 | BIT_30 | BIT_31
      mask Display: fprintf('%s\n%s\n%s',pid_cat,pid_number,bit);
  Constant11 : Constant  Value=0
  wires:
  Constant11/1 -> " "/2(ctrl), " 3"/2(ctrl), " 2"/2(ctrl)
  ccm_iac_mon/1 -> " "/1(data)
  ipsibr/1 -> " 2"/1(data)
  iscflg/1 -> " 3"/1(data)
